simulink model "opg35"  (R2021b)
settings: Solver=FixedStepAuto  StartTime=0.9  StopTime=10  FixedStep=0.02  RelTol=1e-3
settings Model: Creator=klyx  LastModifiedBy=klyx

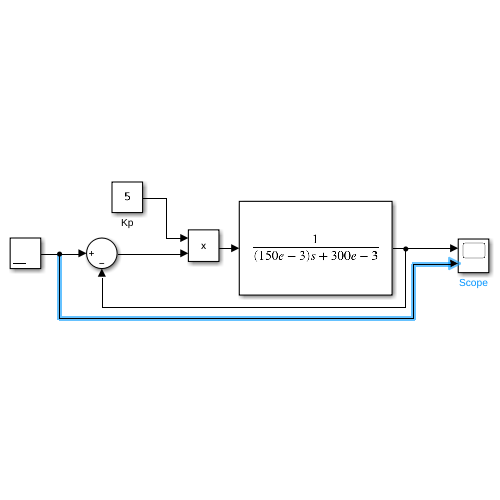
[thumbnail: Simulink's stored preview of the top-level diagram]
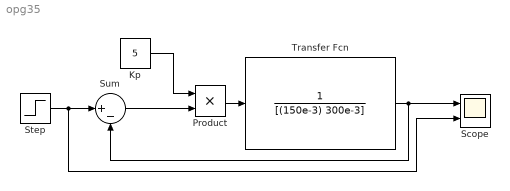
== system opg35 ==
  Kp : Constant  Value=5
  Product : Product
  Scope : Scope  NumInputPorts=2
  Step : Step  SampleTime=0
  Sum : Sum  Inputs=|+-
  Transfer Fcn : TransferFcn  Denominator=[(150e-3) 300e-3]
  wires:
  Step/1 -> Scope/2, Sum/1
  Sum/1 -> Product/2
  Kp/1 -> Product/1
  Transfer Fcn/1 -> Scope/1, Sum/2
  Product/1 -> Transfer Fcn/1
